simulink model "OP"  (R2021a)
settings: Solver=VariableStepAuto  StartTime=0.0  StopTime=10.0  RelTol=1e-3
values from neighbouring files (symbols this model uses):
  kd = eye(3)*4    [params.m]
  kp = eye(3)*10    [params.m]
settings Model: Creator=antoninoparisi  LastModifiedBy=antoninoparisi

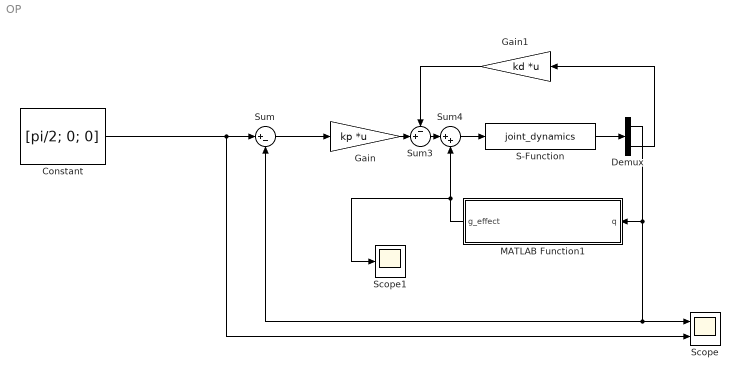
== system OP ==
  Constant : Constant  Value=[pi/2; 0; 0]  VectorParams1D=off
  Demux : Demux  Outputs=2
  Gain : Gain  Gain=kp  Multiplication=Matrix(K*u) (u vector)
  Gain1 : Gain  Gain=kd  Multiplication=Matrix(K*u) (u vector)
  MATLAB Function1 : MATLAB Function  TreatAsAtomicUnit=on
  S-Function : S-Function  FunctionName=joint_dynamics  Parameters=robot  SFunctionDeploymentMode=off  EnableBusSupport=off
  Scope : Scope  NumInputPorts=2
  Scope1 : Scope
  Sum : Sum  Inputs=|+-
  Sum3 : Sum  Inputs=-+|
  Sum4 : Sum  Inputs=|++
  wires:
  Constant/1 -> Sum/1, Scope/2
  S-Function/1 -> Demux/1
  Gain/1 -> Sum3/2
  Gain1/1 -> Sum3/1
  Sum3/1 -> Sum4/1
  Sum4/1 -> S-Function/1
  MATLAB Function1/1(g_effect) -> Sum4/2, Scope1/1
  Demux/2 -> Gain1/1
  Demux/1 -> MATLAB Function1/1(q), Sum/2, Scope/1
  Sum/1 -> Gain/1

== matlab function OP/MATLAB Function1 ==
  data: q input; g_effect output
function g_effect = gravity(q)

g_effect = G_Lagrangian(q);
